simulink model "Aenea_model"  (R2020b)
settings: Solver=FixedStepDiscrete  StartTime=0.0  StopTime=10.0  FixedStep=0.02  RelTol=1e-3
values from neighbouring files (symbols this model uses):
  attuatore_Amax = deg2rad(27)    [AVVIO_AENEA_DATA.m]
  attuatore_Amin = deg2rad(-23)    [AVVIO_AENEA_DATA.m]
  attuatore_Emax = deg2rad(18)    [AVVIO_AENEA_DATA.m]
  attuatore_Emin = deg2rad(-32)    [AVVIO_AENEA_DATA.m]
  attuatore_Rmax = deg2rad(30)    [AVVIO_AENEA_DATA.m]
  attuatore_Rmin = deg2rad(-30)    [AVVIO_AENEA_DATA.m]
  attuatore_Tmax = 1    [AVVIO_AENEA_DATA.m]
  attuatore_Tmin = 0    [AVVIO_AENEA_DATA.m]
  interventoA_05 = 25    [AVVIO_AENEA_DATA.m]
  interventoA_1 = 20    [AVVIO_AENEA_DATA.m]
  interventoE_05 = 20    [AVVIO_AENEA_DATA.m]
  interventoE_1 = 15    [AVVIO_AENEA_DATA.m]
  interventoT = 0.1    [AVVIO_AENEA_DATA.m]
  inv_A = -1    [AVVIO_AENEA_DATA.m]
  inv_comp_h = -1    [AVVIO_AENEA_DATA.m]
  inv_E = 1    [AVVIO_AENEA_DATA.m]
  inv_R = 1    [AVVIO_AENEA_DATA.m]
  inv_T = 1    [AVVIO_AENEA_DATA.m]
  K_AW_B_AP_quota = 1000    [AVVIO_AENEA_DATA.m]
  K_AW_B_becc = -250    [AVVIO_AENEA_DATA.m]
  K_AW_B_imb = 0    [AVVIO_AENEA_DATA.m]
  K_AW_B_roll = 500    [AVVIO_AENEA_DATA.m]
  K_imb_inv = -1    [AVVIO_AENEA_DATA.m]
  Kd_h_app = 0.085    [AVVIO_AENEA_DATA.m]
  Kd_h_flare = 0.01    [AVVIO_AENEA_DATA.m]
  Ki_AP_quota_select = 0.014    [AVVIO_AENEA_DATA.m]
  Ki_AP_rotta = 0.03    [AVVIO_AENEA_DATA.m]
  Ki_AP_vel = 0.001*8    (= 0.008)    [AVVIO_AENEA_DATA.m]
  Ki_becch = -0.064065*10    (= -0.64065)    [AVVIO_AENEA_DATA.m]
  Ki_h_app = 0.055    [AVVIO_AENEA_DATA.m]
  Ki_h_cruise = 0.008    [AVVIO_AENEA_DATA.m]
  Ki_h_flare = 0.07    [AVVIO_AENEA_DATA.m]
  Ki_roll = 0.025*10    (= 0.25)    [AVVIO_AENEA_DATA.m]
  Kp_AP_quota_hold_h = 0.15    [AVVIO_AENEA_DATA.m]
  Kp_AP_quota_hold_l = 1    [AVVIO_AENEA_DATA.m]
  Kp_AP_quota_select = 0.014    [AVVIO_AENEA_DATA.m]
  Kp_AP_rotta = 0.7    [AVVIO_AENEA_DATA.m]
  Kp_AP_vel = 0.2692/8    (= 0.03365)    [AVVIO_AENEA_DATA.m]
  Kp_becch = -0.1918*10    (= -1.918)    [AVVIO_AENEA_DATA.m]
  Kp_comp_h = 0.035*15    (= 0.525)    [AVVIO_AENEA_DATA.m]
  Kp_h_app_max = 0.086    [AVVIO_AENEA_DATA.m]
  Kp_h_app_min = 0.01    [AVVIO_AENEA_DATA.m]
  Kp_h_cruise = 0.04    [AVVIO_AENEA_DATA.m]
  Kp_h_flare = 0.1    [AVVIO_AENEA_DATA.m]
  Kp_imb = -0.04*10    (= -0.4)    [AVVIO_AENEA_DATA.m]
  Kp_p = 0.025*5    (= 0.125)    [AVVIO_AENEA_DATA.m]
  Kp_q = -0.025*5    (= -0.125)    [AVVIO_AENEA_DATA.m]
  Kp_roll = 0.11*10    (= 1.1)    [AVVIO_AENEA_DATA.m]
  Kp_Rotta_ATO = 4    [AVVIO_AENEA_DATA.m]
  phi_max = deg2rad(30)    [AVVIO_AENEA_DATA.m]
  phi_min = deg2rad(-30)    [AVVIO_AENEA_DATA.m]
  pwm_aileron_max = 1940    [AVVIO_AENEA_DATA.m]
  pwm_aileron_min = 1099    [AVVIO_AENEA_DATA.m]
  pwm_elevator_max = 1939    [AVVIO_AENEA_DATA.m]
  pwm_elevator_min = 1099    [AVVIO_AENEA_DATA.m]
  pwm_rudder_max = 1971    [AVVIO_AENEA_DATA.m]
  pwm_rudder_min = 1130    [AVVIO_AENEA_DATA.m]
  pwm_throttle_max = 1940    [AVVIO_AENEA_DATA.m]
  pwm_throttle_min = 1160    [AVVIO_AENEA_DATA.m]
  safe_phi = 55    [AVVIO_AENEA_DATA.m]
  safe_V = 40    [AVVIO_AENEA_DATA.m]
  t_AP = 0.02    [AVVIO_AENEA_DATA.m]
  theta_max = deg2rad(15)    [AVVIO_AENEA_DATA.m]
  theta_min = deg2rad(-15)    [AVVIO_AENEA_DATA.m]
  time_alarm_SAFE = 1    [AVVIO_AENEA_DATA.m]
  V_max = 30    [AVVIO_AENEA_DATA.m]
  V_stall = 11    [AVVIO_AENEA_DATA.m]
  vel_wp1_al = 25    [AVVIO_AENEA_DATA.m]
  vel_wp2_al = 20    [AVVIO_AENEA_DATA.m]
undefined symbols (not defined in the file or in its folder): bias, DiscIntNeverNeededParam, Newton, Q1B, R1B, Raphson, Sensor_Offsets, tsamp, UP, vd_ini
libraries: simulink_extras x41, slpidlib x8, simulink x6, dspsigops x4, arduinolib x3, svdutilitieslib x3, aerolibtransform2sys x2, aerolibtransform2 x2, aerosimlib x2, cstblocks x1
(part 2 of 8)

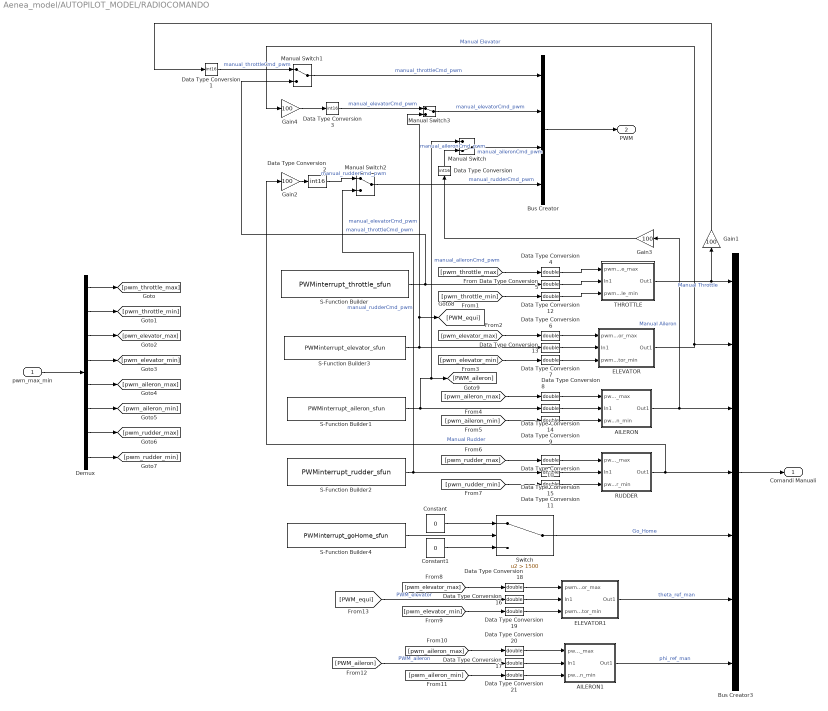
== system Aenea_model/AUTOPILOT_MODEL/RADIOCOMANDO ==
  pwm_max_min : Inport
  AILERON : Subsystem
  AILERON1 : Subsystem
  Bus Creator : BusCreator  Inputs=4
  Bus Creator3 : BusCreator  Inputs=7
  Constant : Constant  Value=0
  Constant1 : Constant  Value=0
  Data Type Conversion{,1..3} (4 alike) : DataTypeConversion  OutDataTypeStr=int16
  Data Type Conversion{4..21} (18 alike) : DataTypeConversion  OutDataTypeStr=double
  Demux : Demux  Outputs=8
  ELEVATOR : Subsystem
  ELEVATOR1 : Subsystem
  Gain{1..4} (4 alike) : Gain  Gain=100
  Manual Switch : ManualSwitch  CurrentSetting=0
  Manual Switch1 : ManualSwitch
  Manual Switch2 : ManualSwitch
  Manual Switch3 : ManualSwitch
  RUDDER : Subsystem
  S-Function Builder : S-Function  FunctionName=PWMinterrupt_throttle_sfun  SFunctionModules=PWMinterrupt_throttle_sfun_wrapper  SFunctionDeploymentMode=off  EnableBusSupport=off  mask(S-Function Builder){}
      mask help: Simulink:masks:SFunctionBuilder_MD
      mask init: same as Aenea_model/LOG_DATA_MODEL/S-Function Builder
      settings: CopyFcn=set_param(gcbh,'LinkStatus','none')  OpenFcn=sfunctionwizard(gcbh)
      mask Display: plot(val(:,1),val(:,2)),disp(sys),port_label('output',1,'out')
  S-Function Builder1 : S-Function  FunctionName=PWMinterrupt_aileron_sfun  SFunctionModules=PWMinterrupt_aileron_sfun_wrapper  SFunctionDeploymentMode=off  EnableBusSupport=off  mask(S-Function Builder){}
      mask help: Simulink:masks:SFunctionBuilder_MD
      mask init: same as Aenea_model/LOG_DATA_MODEL/S-Function Builder
      settings: CopyFcn=set_param(gcbh,'LinkStatus','none')  OpenFcn=sfunctionwizard(gcbh)
      mask Display: plot(val(:,1),val(:,2)),disp(sys),port_label('output',1,'out')
  S-Function Builder2 : S-Function  FunctionName=PWMinterrupt_rudder_sfun  SFunctionModules=PWMinterrupt_rudder_sfun_wrapper  SFunctionDeploymentMode=off  EnableBusSupport=off  mask(S-Function Builder){}
      mask help: Simulink:masks:SFunctionBuilder_MD
      mask init: same as Aenea_model/LOG_DATA_MODEL/S-Function Builder
      settings: CopyFcn=set_param(gcbh,'LinkStatus','none')  OpenFcn=sfunctionwizard(gcbh)
      mask Display: plot(val(:,1),val(:,2)),disp(sys),port_label('output',1,'out')
  S-Function Builder3 : S-Function  FunctionName=PWMinterrupt_elevator_sfun  SFunctionModules=PWMinterrupt_elevator_sfun_wrapper  SFunctionDeploymentMode=off  EnableBusSupport=off  mask(S-Function Builder){}
      mask help: Simulink:masks:SFunctionBuilder_MD
      mask init: same as Aenea_model/LOG_DATA_MODEL/S-Function Builder
      settings: CopyFcn=set_param(gcbh,'LinkStatus','none')  OpenFcn=sfunctionwizard(gcbh)
      mask Display: plot(val(:,1),val(:,2)),disp(sys),port_label('output',1,'out')
  S-Function Builder4 : S-Function  FunctionName=PWMinterrupt_goHome_sfun  SFunctionModules=PWMinterrupt_goHome_sfun_wrapper  SFunctionDeploymentMode=off  EnableBusSupport=off  mask(S-Function Builder){}
      mask help: Simulink:masks:SFunctionBuilder_MD
      mask init: same as Aenea_model/LOG_DATA_MODEL/S-Function Builder
      settings: CopyFcn=set_param(gcbh,'LinkStatus','none')  OpenFcn=sfunctionwizard(gcbh)
      mask Display: plot(val(:,1),val(:,2)),disp(sys),port_label('output',1,'out')
  Switch : Switch  Criteria=u2 > Threshold  Threshold=1500
  THROTTLE : Subsystem
  Comandi Manuali : Outport  VectorParamsAs1DForOutWhenUnconnected=off
  PWM : Outport  Port=2  VectorParamsAs1DForOutWhenUnconnected=off
  wires:
  Bus Creator3/1 -> Comandi Manuali/1
  S-Function Builder4/1 -> Switch/2
  Constant/1 -> Switch/1
  Constant1/1 -> Switch/3
  Switch/1 -> Bus Creator3/5  "Go_Home"
  S-Function Builder2/1 -> Manual Switch2/2, Data Type Conversion15/1  "manual_rudderCmd_pwm"
  S-Function Builder3/1 -> Manual Switch3/2, [PWM_equi], Data Type Conversion13/1  "manual_elevatorCmd_pwm"
  S-Function Builder1/1 -> Data Type Conversion14/1, Manual Switch/1, [PWM_aileron]  "manual_aileronCmd_pwm"
  S-Function Builder/1 -> Manual Switch1/2, Data Type Conversion5/1  "manual_throttleCmd_pwm"
  THROTTLE/1(Out1) -> Gain1/1, Bus Creator3/1  "Manual Throttle"
  ELEVATOR/1(Out1) -> Bus Creator3/2, Gain4/1  "Manual Elevator"
  AILERON/1(Out1) -> Gain3/1, Bus Creator3/3  "Manual Aileron"
  RUDDER/1(Out1) -> Bus Creator3/4, Gain2/1  "Manual Rudder"
  Bus Creator/1 -> PWM/1
  pwm_max_min/1 -> Demux/1
  Demux/1 -> [pwm_throttle_max]
  Demux/2 -> [pwm_throttle_min]
  Demux/3 -> [pwm_elevator_max]
  Demux/4 -> [pwm_elevator_min]
  Demux/5 -> [pwm_aileron_max]
  Demux/6 -> [pwm_aileron_min]
  Demux/8 -> [pwm_rudder_min]
  Demux/7 -> [pwm_rudder_max]
  [pwm_elevator_min] -> Data Type Conversion7/1
  [pwm_elevator_max] -> Data Type Conversion6/1
  [pwm_aileron_min] -> Data Type Conversion9/1
  [pwm_aileron_max] -> Data Type Conversion8/1
  [pwm_rudder_max] -> Data Type Conversion10/1
  [pwm_rudder_min] -> Data Type Conversion11/1
  [pwm_throttle_max] -> Data Type Conversion4/1
  [pwm_throttle_min] -> Data Type Conversion12/1
  Data Type Conversion6/1 -> ELEVATOR/1(pwm_elevator_max)
  Data Type Conversion7/1 -> ELEVATOR/3(pwm_elevator_min)
  Data Type Conversion8/1 -> AILERON/1(pwm_aileron_max)
  Data Type Conversion9/1 -> AILERON/3(pwm_aileron_min)
  Data Type Conversion10/1 -> RUDDER/1(pwm_rudder_max)
  Data Type Conversion11/1 -> RUDDER/3(pwm_rudder_min)
  Data Type Conversion4/1 -> THROTTLE/1(pwm_throttle_max)
  Data Type Conversion5/1 -> THROTTLE/2(In1)
  Data Type Conversion12/1 -> THROTTLE/3(pwm_throttle_min)
  Data Type Conversion13/1 -> ELEVATOR/2(In1)
  Data Type Conversion14/1 -> AILERON/2(In1)
  Data Type Conversion15/1 -> RUDDER/2(In1)
  [pwm_aileron_max] -> Data Type Conversion20/1
  AILERON1/1(Out1) -> Bus Creator3/7  "phi_ref_man"
  [PWM_equi] -> Data Type Conversion16/1  "PWM_elevator"
  ELEVATOR1/1(Out1) -> Bus Creator3/6  "theta_ref_man"
  [pwm_elevator_min] -> Data Type Conversion19/1
  Data Type Conversion17/1 -> AILERON1/2(In1)
  [pwm_aileron_min] -> Data Type Conversion21/1
  Data Type Conversion21/1 -> AILERON1/3(pwm_aileron_min)
  Data Type Conversion18/1 -> ELEVATOR1/1(pwm_elevator_max)
  Data Type Conversion16/1 -> ELEVATOR1/2(In1)
  Data Type Conversion20/1 -> AILERON1/1(pwm_aileron_max)
  Data Type Conversion19/1 -> ELEVATOR1/3(pwm_elevator_min)
  [pwm_elevator_max] -> Data Type Conversion18/1
  [PWM_aileron] -> Data Type Conversion17/1  "PWM_aileron"
  Gain3/1 -> Data Type Conversion/1
  Data Type Conversion/1 -> Manual Switch/2  "manual_aileronCmd_pwm"
  Gain4/1 -> Data Type Conversion3/1
  Data Type Conversion3/1 -> Manual Switch3/1  "manual_elevatorCmd_pwm"
  Data Type Conversion1/1 -> Manual Switch1/1  "manual_throttleCmd_pwm"
  Gain1/1 -> Data Type Conversion1/1
  Gain2/1 -> Data Type Conversion2/1
  Data Type Conversion2/1 -> Manual Switch2/1  "manual_rudderCmd_pwm"
  Manual Switch/1 -> Bus Creator/3  "manual_aileronCmd_pwm"
  Manual Switch1/1 -> Bus Creator/1  "manual_throttleCmd_pwm"
  Manual Switch2/1 -> Bus Creator/4  "manual_rudderCmd_pwm"
  Manual Switch3/1 -> Bus Creator/2  "manual_elevatorCmd_pwm"

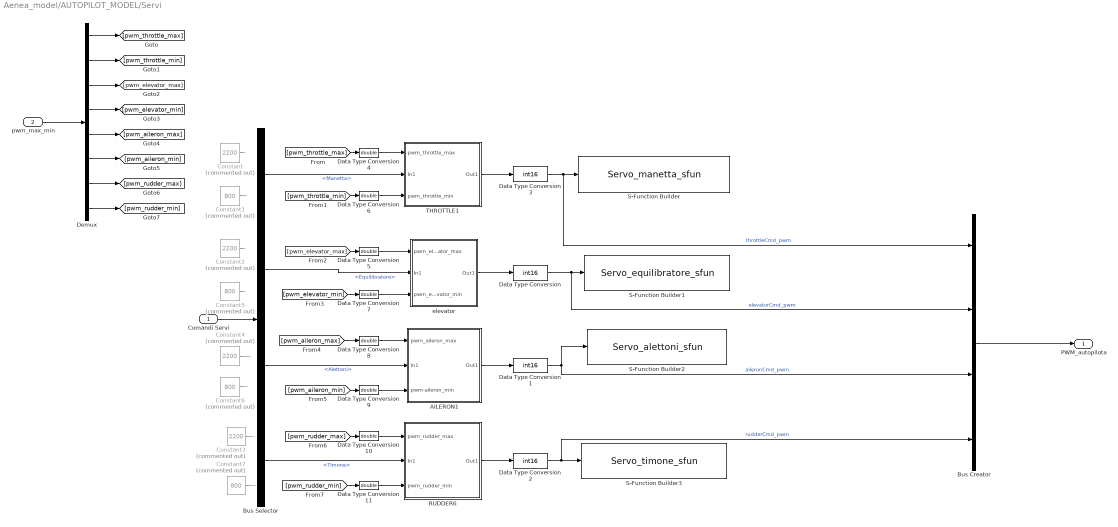
== system Aenea_model/AUTOPILOT_MODEL/Servi ==
  Comandi Servi : Inport
  pwm_max_min : Inport  Port=2
  AILERON1 : Subsystem
  Bus Creator : BusCreator  Inputs=4
  Bus Selector : BusSelector  OutputSignals=Manetta,Equilibratore,Alettoni,Timone
  Constant{,2..4} (4 alike) : Constant  Commented=on  Value=2200
  Constant{1,5..7} (4 alike) : Constant  Commented=on  Value=800
  Data Type Conversion{,1..3} (4 alike) : DataTypeConversion  OutDataTypeStr=int16
  Data Type Conversion{4..11} (8 alike) : DataTypeConversion  OutDataTypeStr=double
  Demux : Demux  Outputs=8
  RUDDER6 : Subsystem
  S-Function Builder : S-Function  FunctionName=Servo_manetta_sfun  SFunctionModules=Servo_manetta_sfun_wrapper  SFunctionDeploymentMode=off  EnableBusSupport=off  mask(S-Function Builder){}
      mask help: Simulink:masks:SFunctionBuilder_MD
      mask init: same as Aenea_model/LOG_DATA_MODEL/S-Function Builder
      settings: CopyFcn=set_param(gcbh,'LinkStatus','none')  OpenFcn=sfunctionwizard(gcbh)
      mask Display:
      | plot(val(:,1),val(:,2))
      | disp(sys)
      | port_label('input',1,'tau')
  S-Function Builder1 : S-Function  FunctionName=Servo_equilibratore_sfun  SFunctionModules=Servo_equilibratore_sfun_wrapper  SFunctionDeploymentMode=off  EnableBusSupport=off  mask(S-Function Builder){}
      mask help: Simulink:masks:SFunctionBuilder_MD
      mask init: same as Aenea_model/LOG_DATA_MODEL/S-Function Builder
      settings: CopyFcn=set_param(gcbh,'LinkStatus','none')  OpenFcn=sfunctionwizard(gcbh)
      mask Display:
      | plot(val(:,1),val(:,2))
      | disp(sys)
      | port_label('input',1,'tau')
  S-Function Builder2 : S-Function  FunctionName=Servo_alettoni_sfun  SFunctionModules=Servo_alettoni_sfun_wrapper  SFunctionDeploymentMode=off  EnableBusSupport=off  mask(S-Function Builder){}
      mask help: Simulink:masks:SFunctionBuilder_MD
      mask init: same as Aenea_model/LOG_DATA_MODEL/S-Function Builder
      settings: CopyFcn=set_param(gcbh,'LinkStatus','none')  OpenFcn=sfunctionwizard(gcbh)
      mask Display:
      | plot(val(:,1),val(:,2))
      | disp(sys)
      | port_label('input',1,'tau')
  S-Function Builder3 : S-Function  FunctionName=Servo_timone_sfun  SFunctionModules=Servo_timone_sfun_wrapper  SFunctionDeploymentMode=off  EnableBusSupport=off  mask(S-Function Builder){}
      mask help: Simulink:masks:SFunctionBuilder_MD
      mask init: same as Aenea_model/LOG_DATA_MODEL/S-Function Builder
      settings: CopyFcn=set_param(gcbh,'LinkStatus','none')  OpenFcn=sfunctionwizard(gcbh)
      mask Display:
      | plot(val(:,1),val(:,2))
      | disp(sys)
      | port_label('input',1,'tau')
  THROTTLE1 : Subsystem
  elevator : Subsystem
  PWM_autopilota : Outport  VectorParamsAs1DForOutWhenUnconnected=off
  wires:
  AILERON1/1(Out1) -> Data Type Conversion1/1
  THROTTLE1/1(Out1) -> Data Type Conversion3/1
  RUDDER6/1(Out1) -> Data Type Conversion2/1
  elevator/1(Out1) -> Data Type Conversion/1
  Bus Selector/1 -> THROTTLE1/2(In1)  "<Manetta>"
  Bus Selector/4 -> RUDDER6/2(In1)  "<Timone>"
  Bus Selector/3 -> AILERON1/2(In1)  "<Alettoni>"
  Bus Selector/2 -> elevator/2(In1)  "<Equilibratore>"
  Comandi Servi/1 -> Bus Selector/1
  Demux/3 -> [pwm_elevator_max]
  Demux/2 -> [pwm_throttle_min]
  Demux/6 -> [pwm_aileron_min]
  Demux/1 -> [pwm_throttle_max]
  Demux/8 -> [pwm_rudder_min]
  Demux/7 -> [pwm_rudder_max]
  Demux/5 -> [pwm_aileron_max]
  Demux/4 -> [pwm_elevator_min]
  [pwm_throttle_max] -> Data Type Conversion4/1
  [pwm_throttle_min] -> Data Type Conversion6/1
  [pwm_elevator_max] -> Data Type Conversion5/1
  [pwm_elevator_min] -> Data Type Conversion7/1
  [pwm_aileron_max] -> Data Type Conversion8/1
  [pwm_aileron_min] -> Data Type Conversion9/1
  [pwm_rudder_max] -> Data Type Conversion10/1
  Data Type Conversion/1 -> S-Function Builder1/1, Bus Creator/2  "elevatorCmd_pwm"
  Data Type Conversion1/1 -> S-Function Builder2/1, Bus Creator/3  "aileronCmd_pwm"
  Data Type Conversion3/1 -> S-Function Builder/1, Bus Creator/1  "throttleCmd_pwm"
  Data Type Conversion2/1 -> S-Function Builder3/1, Bus Creator/4  "rudderCmd_pwm"
  Data Type Conversion4/1 -> THROTTLE1/1(pwm_throttle_max)
  Data Type Conversion6/1 -> THROTTLE1/3(pwm_throttle_min)
  Data Type Conversion5/1 -> elevator/1(pwm_elevator_max)
  Data Type Conversion7/1 -> elevator/3(pwm_elevator_min)
  Data Type Conversion8/1 -> AILERON1/1(pwm_aileron_max)
  Data Type Conversion9/1 -> AILERON1/3(pwm-aileron_min)
  Data Type Conversion10/1 -> RUDDER6/1(pwm_rudder_max)
  Data Type Conversion11/1 -> RUDDER6/3("pwm_rudder_min ")
  Bus Creator/1 -> PWM_autopilota/1
  Constant1/1 -> ?
  Constant/1 -> ?
  Constant2/1 -> ?
  Constant3/1 -> ?
  Constant4/1 -> ?
  Constant5/1 -> ?
  Constant6/1 -> ?
  Constant7/1 -> ?
  pwm_max_min/1 -> Demux/1
  [pwm_rudder_min] -> Data Type Conversion11/1

== system Aenea_model/LOG_DATA_MODEL/LOG_BOOL_SIGNALS ==
  dummy16 : Inport
  Bus Creator11 : BusCreator  Inputs=2  OutDataTypeStr=Bus: BUS_bool_log_t  NonVirtualBus=on
      settings: InheritFromInputs=off
  Constant24 : Constant  Value=true  OutDataTypeStr=boolean
  bool_data : Outport
  wires:
  Constant24/1 -> Bus Creator11/1  "dummy12"
  Bus Creator11/1 -> bool_data/1  "bool_data"
  dummy16/1 -> Bus Creator11/2

== system Aenea_model/LOG_DATA_MODEL/LOG_DOUBLE_SIGNALS ==
  double_in : Inport
  Bus Creator : BusCreator  Inputs=8
  Bus Selector : BusSelector  OutputSignals=sensor_data_raw.Lat,sensor_data_raw.Long,sensor_data_filtered.Lat,sensor_data_filtered.Long,absDelta.absE,absDelta.absA,absDelta.absT
  Mux : Mux  Inputs=1
  Mux1 : Mux  Inputs=1
  Radians to Degrees : simulink_extras/Transformations/Radians to Degrees
  Radians to Degrees1 : simulink_extras/Transformations/Radians to Degrees
  Subsystem : Subsystem
  double_data : Outport
  wires:
  Bus Creator/1 -> double_data/1  "double_data"
  Subsystem/1(frame_count) -> Bus Creator/1  "time_frame"
  double_in/1 -> Bus Selector/1
  Bus Selector/1 -> Mux/1  "<Lat>"
  Bus Selector/2 -> Mux1/1  "<Long>"
  Bus Selector/3 -> Radians to Degrees/1  "<Lat>"
  Bus Selector/4 -> Radians to Degrees1/1  "<Long>"
  Mux/1 -> Bus Creator/2  "Lat_raw"
  Mux1/1 -> Bus Creator/3  "Long_raw"
  Radians to Degrees/1 -> Bus Creator/4  "Lat"
  Radians to Degrees1/1 -> Bus Creator/5  "Long"
  Bus Selector/5 -> Bus Creator/6  "<absE>"
  Bus Selector/6 -> Bus Creator/7  "<absA>"
  Bus Selector/7 -> Bus Creator/8  "<absT>"

== system Aenea_model/LOG_DATA_MODEL/LOG_INT16_SIGNALS ==
  int16_in : Inport
  Bus Creator7 : BusCreator  Inputs=8  OutDataTypeStr=Bus: BUS_int16_log_t  NonVirtualBus=on
      settings: InheritFromInputs=off
  Bus Selector : BusSelector  OutputSignals=sensor_data_raw.Comandi.manual_throttleCmd_pwm,sensor_data_raw.Comandi.manual_elevatorCmd_pwm,sensor_data_raw.Comandi.manual_aileronCmd_pwm,sensor_data_raw.Comandi.manual_rudderCmd_pwm,sensor_data_raw.PWM_autopilota.throttleCmd_pwm,sensor_data_raw.PWM_autopilota.elevatorCmd_pwm,sensor_data_raw.PWM_autopilota.aileronCmd_pwm,sensor_data_raw.PWM_autopilota.rudderCmd_pwm
  int16_data : Outport
  wires:
  Bus Creator7/1 -> int16_data/1  "int16_data"
  int16_in/1 -> Bus Selector/1
  Bus Selector/1 -> Bus Creator7/1  "<manual_throttleCmd_pwm>"
  Bus Selector/2 -> Bus Creator7/2  "<manual_elevatorCmd_pwm>"
  Bus Selector/3 -> Bus Creator7/3  "<manual_aileronCmd_pwm>"
  Bus Selector/4 -> Bus Creator7/4  "<manual_rudderCmd_pwm>"
  Bus Selector/5 -> Bus Creator7/5  "<throttleCmd_pwm>"
  Bus Selector/6 -> Bus Creator7/6  "<elevatorCmd_pwm>"
  Bus Selector/7 -> Bus Creator7/7  "<aileronCmd_pwm>"
  Bus Selector/8 -> Bus Creator7/8  "<rudderCmd_pwm>"

== system Aenea_model/LOG_DATA_MODEL/LOG_INT32_SIGNALS ==
  Bus Creator5 : BusCreator  Inputs=2  OutDataTypeStr=Bus: BUS_int32_log_t  NonVirtualBus=on
      settings: InheritFromInputs=off
  Constant18 : Constant  Value=-15  OutDataTypeStr=int32
  Constant9 : Constant  Value=528  OutDataTypeStr=int32
  int32_data : Outport
  wires:
  Constant18/1 -> Bus Creator5/2  "dummy4"
  Bus Creator5/1 -> int32_data/1  "int32_data"
  Constant9/1 -> Bus Creator5/1  "dummy3"

== system Aenea_model/LOG_DATA_MODEL/LOG_INT8_SIGNALS ==
  IN_LOG : Inport
  Bus Creator9 : BusCreator  Inputs=2  OutDataTypeStr=Bus: BUS_int8_log_t  NonVirtualBus=on
      settings: InheritFromInputs=off
  Bus Selector : BusSelector  OutputSignals=modo.modo,go_home
  Data Type Conversion : DataTypeConversion  OutDataTypeStr=int8
  Data Type Conversion1 : DataTypeConversion  OutDataTypeStr=int8
  int8_data : Outport
  wires:
  IN_LOG/1 -> Bus Selector/1
  Bus Creator9/1 -> int8_data/1  "int8_data"
  Bus Selector/1 -> Data Type Conversion/1  "<modo>"
  Data Type Conversion/1 -> Bus Creator9/1
  Bus Selector/2 -> Data Type Conversion1/1  "<go_home>"
  Data Type Conversion1/1 -> Bus Creator9/2

== system Aenea_model/LOG_DATA_MODEL/LOG_SINGLE_SIGNALS ==
  single_in : Inport
  Bus Creator4 : BusCreator  Inputs=24  OutDataTypeStr=Bus: BUS_single_log_t  NonVirtualBus=on
      settings: InheritFromInputs=off
  Bus Selector : BusSelector  OutputSignals=sensor_data_raw.V_GPS,sensor_data_raw.quota_GPS,sensor_data_raw.heading,sensor_data_raw.acc x,sensor_data_raw.acc y,sensor_data_raw.acc z,sensor_data_raw.p,sensor_data_raw.q,sensor_data_raw.r,sensor_data_raw.phi,sensor_data_raw.theta,sensor_data_raw.psi,sensor_data_raw.V_pitot,sensor_data_raw.dist_lidar,sensor_data_raw.quota_baro,sensor_data_raw.pressione,sensor_data_raw.temperatura,sensor_data_filtered.Alt,sensor_data_filtered.ias,sensor_data_filtered.RC,sensor_data_filtered.horiz_speed,sensor_data_filtered.heading,sensor_data_filtered.quota_lidar,dp
  Data Type Conversion{,1..23} (24 alike) : DataTypeConversion  OutDataTypeStr=single
  single_data : Outport
  wires:
  Bus Creator4/1 -> single_data/1  "single_data"
  single_in/1 -> Bus Selector/1
  Bus Selector/2 -> Data Type Conversion1/1  "<quota_GPS>"
  Bus Selector/1 -> Data Type Conversion/1  "<V_GPS>"
  Bus Selector/3 -> Data Type Conversion2/1  "<heading>"
  Bus Selector/4 -> Data Type Conversion3/1  "<acc x>"
  Bus Selector/5 -> Data Type Conversion4/1  "<acc y>"
  Bus Selector/6 -> Data Type Conversion5/1  "<acc z>"
  Bus Selector/7 -> Data Type Conversion6/1  "<p>"
  Bus Selector/8 -> Data Type Conversion7/1  "<q>"
  Bus Selector/9 -> Data Type Conversion8/1  "<r>"
  Bus Selector/11 -> Data Type Conversion9/1  "<theta>"
  Bus Selector/12 -> Data Type Conversion10/1  "<psi>"
  Bus Selector/13 -> Data Type Conversion11/1  "<V_pitot>"
  Bus Selector/14 -> Data Type Conversion12/1  "<dist_lidar>"
  Data Type Conversion/1 -> Bus Creator4/1  "v_gps_raw"
  Data Type Conversion1/1 -> Bus Creator4/2  "h_gps_raw"
  Data Type Conversion2/1 -> Bus Creator4/3  "heading_raw"
  Data Type Conversion3/1 -> Bus Creator4/4  "acc_x_raw"
  Data Type Conversion5/1 -> Bus Creator4/6  "acc_z_raw"
  Data Type Conversion6/1 -> Bus Creator4/7  "p_raw"
  Data Type Conversion7/1 -> Bus Creator4/8  "q_raw"
  Data Type Conversion4/1 -> Bus Creator4/5  "acc_y_raw"
  Data Type Conversion8/1 -> Bus Creator4/9  "r_raw"
  Data Type Conversion10/1 -> Bus Creator4/12  "psi_raw"
  Data Type Conversion9/1 -> Bus Creator4/11  "theta_raw"
  Data Type Conversion11/1 -> Bus Creator4/13  "v_pitot_raw"
  Data Type Conversion12/1 -> Bus Creator4/14  "dist_lidar_raw"
  Bus Selector/10 -> Data Type Conversion13/1  "<phi>"
  Data Type Conversion13/1 -> Bus Creator4/10  "phi_raw"
  Bus Selector/18 -> Data Type Conversion18/1  "<Alt>"
  Bus Selector/19 -> Data Type Conversion17/1  "<ias>"
  Bus Selector/20 -> Data Type Conversion19/1  "<RC>"
  Bus Selector/21 -> Data Type Conversion14/1  "<horiz_speed>"
  Bus Selector/22 -> Data Type Conversion15/1  "<heading>"
  Bus Selector/23 -> Data Type Conversion16/1  "<quota_lidar>"
  Data Type Conversion18/1 -> Bus Creator4/18  "h_baro_filt"
  Data Type Conversion17/1 -> Bus Creator4/19  "ias_filt"
  Data Type Conversion19/1 -> Bus Creator4/20  "RC_filt"
  Data Type Conversion14/1 -> Bus Creator4/21  "groundspeed_filt"
  Data Type Conversion15/1 -> Bus Creator4/22  "heading_filt"
  Data Type Conversion16/1 -> Bus Creator4/23  "dist_lidar_filt"
  Bus Selector/15 -> Data Type Conversion20/1  "<quota_baro>"
  Bus Selector/16 -> Data Type Conversion21/1  "<pressione>"
  Bus Selector/17 -> Data Type Conversion22/1  "<temperatura>"
  Data Type Conversion20/1 -> Bus Creator4/15  "h_baro_raw"
  Data Type Conversion21/1 -> Bus Creator4/16  "press_raw"
  Data Type Conversion22/1 -> Bus Creator4/17  "temp_raw"
  Bus Selector/24 -> Data Type Conversion23/1  "<dp>"
  Data Type Conversion23/1 -> Bus Creator4/24  "dp_raw"

== system Aenea_model/LOG_DATA_MODEL/LOG_UINT16_SIGNALS ==
  Bus Creator8 : BusCreator  Inputs=2  OutDataTypeStr=Bus: BUS_uint16_log_t  NonVirtualBus=on
      settings: InheritFromInputs=off
  Constant11 : Constant  Value=20  OutDataTypeStr=uint16
  Constant22 : Constant  Value=20  OutDataTypeStr=uint16
  uint16_data : Outport
  wires:
  Bus Creator8/1 -> uint16_data/1  "uint16_data"
  Constant22/1 -> Bus Creator8/2  "dummy10"
  Constant11/1 -> Bus Creator8/1  "dummy9"

== system Aenea_model/LOG_DATA_MODEL/LOG_UINT32_SIGNALS ==
  Bus Creator6 : BusCreator  Inputs=2  OutDataTypeStr=Bus: BUS_uint32_log_t  NonVirtualBus=on
      settings: InheritFromInputs=off
  Constant19 : Constant  Value=15  OutDataTypeStr=uint32
  Constant20 : Constant  Value=1078  OutDataTypeStr=uint32
  uint32_data : Outport
  wires:
  Constant20/1 -> Bus Creator6/2  "dummy6"
  Constant19/1 -> Bus Creator6/1  "dummy5"
  Bus Creator6/1 -> uint32_data/1  "uint32_data"

== system Aenea_model/LOG_DATA_MODEL/LOG_UINT8_SIGNALS ==
  uint8_in : Inport
  Bus Creator : BusCreator  Inputs=2
  Bus Selector : BusSelector  OutputSignals=sensor_data_raw.fix,Base_mode
  Data Type Conversion : DataTypeConversion  OutDataTypeStr=uint8
  Data Type Conversion1 : DataTypeConversion  OutDataTypeStr=uint8
  uint8_data : Outport
  wires:
  Data Type Conversion/1 -> Bus Creator/1  "gps_fix"
  uint8_in/1 -> Bus Selector/1
  Bus Creator/1 -> uint8_data/1  "uint8_data"
  Bus Selector/1 -> Data Type Conversion/1  "<fix>"
  Bus Selector/2 -> Data Type Conversion1/1  "<Base_mode>"
  Data Type Conversion1/1 -> Bus Creator/2  "Base_mode"

== system Aenea_model/AUTOPILOT_MODEL/AIR TX/Enable  ==
  In1 : Inport
  In2 : Inport  Port=2
  Enable : EnablePort
  Chart : Stateflow chart  TreatAsAtomicUnit=on
  wires:
  In2/1 -> Chart/2(Len)
  In1/1 -> Chart/1(datain)

== system Aenea_model/AUTOPILOT_MODEL/AIR TX/GPS ==
  note: NB.: se non si posside un dato inserire una costante con valore 0. I dati vanno messi tutti anche se zeri nell'ordine elencato
  note: Vanno inseriti i collegamenti con i dati provenienti dal sensore GPS
      | in uscita bisogna dare 3 segnali:
      |
      | -LLAA: latitudine, longitudine, altitudine, altitudine relativa
      | -VEL: velocità (x,y,z)
      | -HDG: heading
  GPS1 : Inport
  Bus Selector : BusSelector  OutputSignals=Lat,Long,Alt,horiz_speed,RC,heading
  Data Type Conversion : DataTypeConversion  OutDataTypeStr=int32  RndMeth=Simplest
  Data Type Conversion1 : DataTypeConversion  OutDataTypeStr=int16  RndMeth=Simplest
  Data Type Conversion2 : DataTypeConversion  OutDataTypeStr=uint16  RndMeth=Simplest
  Gain : Gain  Gain=[10^7;10^7;1000 ;1000]
  Gain1 : Gain  Gain=1000
  Gain2 : Gain  Gain=100
  Mux : Mux
  Mux1 : Mux  Inputs=3
  Radians to Degrees : simulink_extras/Transformations/Radians to Degrees
  Radians to Degrees2 : simulink_extras/Transformations/Radians to Degrees
  alt_r : Constant  Value=0
  vel y : Constant  Value=0  OutDataTypeStr=double
  LLAA : Outport  VectorParamsAs1DForOutWhenUnconnected=off
  vel : Outport  Port=2  VectorParamsAs1DForOutWhenUnconnected=off
  hdg1 : Outport  Port=3  VectorParamsAs1DForOutWhenUnconnected=off
  wires:
  Gain2/1 -> Data Type Conversion2/1
  Gain/1 -> Data Type Conversion/1
  Gain1/1 -> Data Type Conversion1/1
  Mux/1 -> Gain/1
  Bus Selector/6 -> Gain2/1  "<heading>"
  Bus Selector/5 -> Mux1/3  "<RC>"
  Mux1/1 -> Gain1/1  "VEL"
  alt_r/1 -> Mux/4
  GPS1/1 -> Bus Selector/1
  Bus Selector/1 -> Radians to Degrees/1  "<Lat>"
  Bus Selector/2 -> Radians to Degrees2/1  "<Long>"
  Bus Selector/4 -> Mux1/1  "<horiz_speed>"
  vel y/1 -> Mux1/2
  Data Type Conversion2/1 -> hdg1/1
  Data Type Conversion1/1 -> vel/1
  Data Type Conversion/1 -> LLAA/1
  Bus Selector/3 -> Mux/3  "<Alt>"
  Radians to Degrees/1 -> Mux/1  "Lat"
  Radians to Degrees2/1 -> Mux/2  "Long"

== system Aenea_model/AUTOPILOT_MODEL/AIR TX/Heartbeat ==
  note: Vanno inseriti i collegamenti con i dati provenienti dalla ricezione (stazione di terra) e gli allarmi
      | in uscita bisogna dare 2 vettori costituiti da:
      | -I:
      | -custom code (su può mettere ciò che si vuole)
      | -II:
      | -vettore di 2 componenti: tido di veivolo e tipo di autopilota
      | -vettore di due componenti che è creato tramite la matlabfuncition
  Alarm : Inport
  RX_mode : Inport  Port=2
  modo : Inport  Port=3
  Alarm set : MATLAB Function  TreatAsAtomicUnit=on
  Data Type Conversion : DataTypeConversion  OutDataTypeStr=uint32
  Data Type Conversion1 : DataTypeConversion  OutDataTypeStr=uint8
  Mux : Mux  Inputs=2
  Type fixed_wing Autopilot generic : Constant  Value=[1;0]  OutDataTypeStr=uint8
  custom : Outport  VectorParamsAs1DForOutWhenUnconnected=off
  H_data : Outport  Port=2  VectorParamsAs1DForOutWhenUnconnected=off
  wires:
  modo/1 -> Data Type Conversion/1
  Data Type Conversion1/1 -> H_data/1
  Data Type Conversion/1 -> custom/1
  RX_mode/1 -> Alarm set/2(Rx_mode)
  Alarm/1 -> Alarm set/1(Alarm)
  Type fixed_wing Autopilot generic/1 -> Mux/1
  Alarm set/1(H_mav) -> Mux/2
  Mux/1 -> Data Type Conversion1/1

== system Aenea_model/AUTOPILOT_MODEL/AIR TX/IMU & Attidude ==
  note: NB.: se non si posside un dato inserire una costante con valore 0. I dati vanno messi tutti anche se zeri nell'ordine elencato
  note: Vanno inseriti i collegamenti con i dati provenienti dal sensore inerziale (MTi)
      | in uscita bisogna dare un vettore di 12 componenti contente in ordine:
      | - 3 accelerazioni (x,y,z)
      | - 3 giroscopiche (p,q,r)
      | - 3 comp. campo magnetico
      | -3 angoli di eulero
  AHRS1 : Inport
  Bus Selector : BusSelector  OutputSignals=acc,p,q,r,phi,theta,psi
  Constant : Constant  Value=0  OutDataTypeStr=double  SampleTime=t_AP
  Constant1 : Constant  Value=0  OutDataTypeStr=double  SampleTime=t_AP
  Constant2 : Constant  Value=0  OutDataTypeStr=double  SampleTime=t_AP
  Data Type Conversion : DataTypeConversion  OutDataTypeStr=int16  RndMeth=Simplest
  Data Type Conversion1 : DataTypeConversion  OutDataTypeStr=single
  Gain : Gain  Gain=10^3
  Mux{1,3..5} (4 alike) : Mux  Inputs=3
  Mux2 : Mux  Inputs=2
  IMU : Outport  VectorParamsAs1DForOutWhenUnconnected=off
  ATT : Outport  Port=2  VectorParamsAs1DForOutWhenUnconnected=off
  wires:
  Constant/1 -> Mux5/1
  Mux4/1 -> Mux2/1
  Bus Selector/7 -> Mux4/3  "<psi>"
  Bus Selector/6 -> Mux4/2  "<theta>"
  Bus Selector/5 -> Mux4/1  "<phi>"
  Mux3/1 -> Mux2/2, Mux1/2
  Bus Selector/4 -> Mux3/3  "<r>"
  Bus Selector/3 -> Mux3/2  "<q>"
  Bus Selector/2 -> Mux3/1  "<p>"
  Bus Selector/1 -> Mux1/1  "<acc>"
  AHRS1/1 -> Bus Selector/1
  Mux2/1 -> Data Type Conversion1/1
  Gain/1 -> Data Type Conversion/1
  Data Type Conversion1/1 -> ATT/1
  Data Type Conversion/1 -> IMU/1
  Mux1/1 -> Gain/1
  Constant1/1 -> Mux5/2
  Mux5/1 -> Mux1/3
  Constant2/1 -> Mux5/3

== system Aenea_model/AUTOPILOT_MODEL/AIR TX/If_subsystem ==
  note: Blocco per la temporizzazione dell'invio dei messaggi
  Data Type Conversion3 : DataTypeConversion  OutDataTypeStr=uint32  RndMeth=Simplest
  Gain : Gain  Gain=100
  Subsystem : Subsystem
  iflogic_function : MATLAB Function  TreatAsAtomicUnit=on
  iflogic : Outport  VectorParamsAs1DForOutWhenUnconnected=off
  time : Outport  Port=2  VectorParamsAs1DForOutWhenUnconnected=off
  wires:
  Subsystem/3(time) -> Gain/1
  Subsystem/2(H_10) -> iflogic_function/2(H10)
  Subsystem/1(H_50) -> iflogic_function/1(H50)
  Gain/1 -> Data Type Conversion3/1
  Data Type Conversion3/1 -> time/1
  iflogic_function/1(iflogic) -> iflogic/1

== system Aenea_model/AUTOPILOT_MODEL/AIR TX/Servo ==
  note: NB.: se non si posside un dato inserire una costante con valore 0. I dati vanno messi tutti anche se zeri nell'ordine elencato
  note: Vanno inseriti i collegamenti con i dati provenienti dal sensore di velocità
      | in uscita bisogna dare 1 segnale composto da:
      |
      | -  PORT
      | -8 servo
  note: La quota lidar la invio come componente 8 dei servi
  Sensor : Inport
  Servo : Inport  Port=2
  Bus Selector : BusSelector  OutputSignals=Manetta,Equilibratore,Alettoni,Timone
  Bus Selector1 : BusSelector  OutputSignals=quota_lidar
  Constant : Constant  Value=4
  Constant1 : Constant  Value=zeros(3,1)
  Conversione : Subsystem
  Data Type Conversion1 : DataTypeConversion  OutDataTypeStr=uint16  RndMeth=Simplest
  Gain : Gain  Gain=100
  Mux : Mux  Inputs=7
  Saturation : Saturate  UpperLimit=4000  LowerLimit=0
  Servo_data : Outport  VectorParamsAs1DForOutWhenUnconnected=off
  wires:
  Conversione/4(Out4) -> Mux/5
  Conversione/3(Out3) -> Mux/4
  Conversione/2(Out2) -> Mux/3
  Conversione/1(Out1) -> Mux/2
  Bus Selector/1 -> Conversione/1(Manetta)  "<Manetta>"
  Bus Selector/4 -> Conversione/4(Timone)  "<Timone>"
  Bus Selector/3 -> Conversione/3(Alettoni)  "<Alettoni>"
  Bus Selector/2 -> Conversione/2(Equilibratore)  "<Equilibratore>"
  Constant1/1 -> Mux/6
  Constant/1 -> Mux/1
  Servo/1 -> Bus Selector/1
  Mux/1 -> Data Type Conversion1/1
  Data Type Conversion1/1 -> Servo_data/1  "Heading"
  Sensor/1 -> Bus Selector1/1
  Bus Selector1/1 -> Gain/1  "<quota_lidar>"
  Gain/1 -> Saturation/1
  Saturation/1 -> Mux/7

== system Aenea_model/AUTOPILOT_MODEL/AIR TX/Subsystem ==
  In1 : Inport
  In2 : Inport  Port=2
  Enable : EnablePort
  S-Function Builder : S-Function  FunctionName=MavLink_Send_sfun  SFunctionModules=MavLink_Send_sfun_wrapper  SFunctionDeploymentMode=off  EnableBusSupport=off  mask(S-Function Builder){}
      mask help: Simulink:masks:SFunctionBuilder_MD
      mask init: same as Aenea_model/LOG_DATA_MODEL/S-Function Builder
      settings: CopyFcn=set_param(gcbh,'LinkStatus','none')  OpenFcn=sfunctionwizard(gcbh)
      mask Display: plot(val(:,1),val(:,2)),disp(sys),port_label('input',1,'mavlink_buf_out'),port_label('input',2,'mavlink_buf_len')
  wires:
  In1/1 -> S-Function Builder/1
  In2/1 -> S-Function Builder/2

== system Aenea_model/AUTOPILOT_MODEL/AIR TX/SystemStatus ==
  note: coefficiente moltiplicativo Mavlink
  note: conversione
      | Amper - milliAmper
  note: NB.: se non si posside un dato inserire una costante con valore 0 (se non indicato diversamente sopra).
      | I dati vanno messi tutti anche se zeri nell'ordine elencato
  note: Vanno inseriti i collegamenti con i dati provenienti dal autopilota
      | in uscita bisogna dare 4 segnali:
      |
      | -onboard_control_sensor_present
      | - vettore con: load, voltaggio batteria(millivolt), drop rate, 5 flag di errore
      | -corrente della batteria (10*milliamper) -1 se non noto
      | -batteria rimanente (in percentuale) -1 se non noto
  note: conversione
      | Amper - milliAmper
  SyS_input : Inport
  Alarm : Inport  Port=2
  batteria : Inport  Port=3
  " " : Constant  Value=0  OutDataTypeStr=uint16
  Data Type Conversion : DataTypeConversion  OutDataTypeStr=uint32
  Data Type Conversion1 : DataTypeConversion  OutDataTypeStr=int16
  Data Type Conversion2 : DataTypeConversion  OutDataTypeStr=uint16
  Data Type Conversion3 : DataTypeConversion  OutDataTypeStr=int8
  Data Type Conversion4 : DataTypeConversion  OutDataTypeStr=uint16
  Demux : Demux  Outputs=3
  Gain : Gain  Gain=1000  OutDataTypeStr=uint16
  Gain1 : Gain  Gain=0.1  OutDataTypeStr=int16
  Gain2 : Gain  Gain=1000  OutDataTypeStr=int16
  Mux : Mux  Inputs=5
  load uint16 : Constant  Value=10  OutDataTypeStr=uint16
  onboard_control_sensor_present uint32 : Constant  Value=[1; 1 ;1]  OutDataTypeStr=uint32
  onboard : Outport  VectorParamsAs1DForOutWhenUnconnected=off
  LVDE : Outport  Port=2  VectorParamsAs1DForOutWhenUnconnected=off
  B_current : Outport  Port=3  VectorParamsAs1DForOutWhenUnconnected=off
  B_remaining : Outport  Port=4  VectorParamsAs1DForOutWhenUnconnected=off
  wires:
  Gain2/1 -> Gain1/1
  Demux/3 -> Gain2/1
  Gain1/1 -> Data Type Conversion1/1
  Demux/1 -> Gain/1
  batteria/1 -> Demux/1
  " "/1 -> Mux/4
  Data Type Conversion4/1 -> Mux/5
  Alarm/1 -> Data Type Conversion4/1
  SyS_input/1 -> Mux/3
  Data Type Conversion3/1 -> B_remaining/1  "B_Remaining"
  Data Type Conversion1/1 -> B_current/1  "B_Current"
  Data Type Conversion2/1 -> LVDE/1  "LVDE"
  Data Type Conversion/1 -> onboard/1  "onboard"
  Demux/2 -> Data Type Conversion3/1
  Mux/1 -> Data Type Conversion2/1
  Gain/1 -> Mux/2
  load uint16/1 -> Mux/1
  onboard_control_sensor_present uint32/1 -> Data Type Conversion/1

== system Aenea_model/AUTOPILOT_MODEL/AIR TX/VFR ==
  note: NB.: se non si posside un dato inserire una costante con valore 0. I dati vanno messi tutti anche se zeri nell'ordine elencato
  note: Vanno inseriti i collegamenti con i dati provenienti dal sensore di velocità
      | in uscita bisogna dare 3 segnali:
      |
      | -  AGAC: airspeed, groundspeed,altitudine, rateo salita
      | -Heading
      | -Throttle: spinta o rpm del motore
  note: inserire 100/massimo valore
      | deve uscire una percentuale
      | FISSATO PER QUOTA IL 5-5-2016
  VFR1 : Inport
  Bus Selector : BusSelector  OutputSignals=ias,Alt,RC,heading,RPM
  Data Type Conversion : DataTypeConversion  OutDataTypeStr=single
  Data Type Conversion1 : DataTypeConversion  OutDataTypeStr=int16  RndMeth=Simplest
  Data Type Conversion2 : DataTypeConversion  OutDataTypeStr=uint16  RndMeth=Simplest
  Mux : Mux
  Radians to Degrees : simulink_extras/Transformations/Radians to Degrees
  USCITA PERCENTUALE : Gain  Gain=100/9000
  airspeed groundspeed alt climb1 : Constant  Value=0  OutDataTypeStr=double  SampleTime=t_AP
  wrapTo360 : Subsystem
  AGAC : Outport  VectorParamsAs1DForOutWhenUnconnected=off
  Heading : Outport  Port=2  VectorParamsAs1DForOutWhenUnconnected=off
  Throttle : Outport  Port=3  VectorParamsAs1DForOutWhenUnconnected=off
  wires:
  Mux/1 -> Data Type Conversion/1
  Bus Selector/5 -> USCITA PERCENTUALE/1  "<RPM>"
  Bus Selector/4 -> Radians to Degrees/1  "<heading>"
  Bus Selector/3 -> Mux/4  "<RC>"
  Bus Selector/2 -> Mux/3  "<Alt>"
  Bus Selector/1 -> Mux/1  "<ias>"
  airspeed groundspeed alt climb1/1 -> Mux/2
  VFR1/1 -> Bus Selector/1
  Data Type Conversion2/1 -> Throttle/1  "Throttle"
  Data Type Conversion1/1 -> Heading/1  "Heading"
  Data Type Conversion/1 -> AGAC/1  "AGAC"
  USCITA PERCENTUALE/1 -> Data Type Conversion2/1
  Radians to Degrees/1 -> wrapTo360/1(In1)
  wrapTo360/1(Out1) -> Data Type Conversion1/1  "uscita"

== system Aenea_model/AUTOPILOT_MODEL/AIR TX/Waypoints ==
  GC_req : Inport
  "Sensori " : Inport  Port=2
  Bus Selector : BusSelector  OutputSignals=Alt
  Bus Selector3 : BusSelector  OutputSignals=Val_float,WP_db_info,WP_db_param,GC_info
  MATLAB Function : MATLAB Function  TreatAsAtomicUnit=on
  Terminator : Terminator
  GC_info : Outport  VectorParamsAs1DForOutWhenUnconnected=off
  P_value : Outport  Port=2  VectorParamsAs1DForOutWhenUnconnected=off
  WP_info : Outport  Port=3  VectorParamsAs1DForOutWhenUnconnected=off
  WP_param : Outport  Port=4  VectorParamsAs1DForOutWhenUnconnected=off
  wires:
  "Sensori "/1 -> Bus Selector/1
  Bus Selector3/1 -> P_value/1  "<Val_float>"
  Bus Selector/1 -> Terminator/1  "<Alt>"
  MATLAB Function/2(WP_param) -> WP_param/1
  Bus Selector3/3 -> MATLAB Function/2(WP_param_in)  "<WP_db_param>"
  MATLAB Function/1(WP_info) -> WP_info/1
  Bus Selector3/2 -> MATLAB Function/1(WP_info_in)  "<WP_db_info>"
  Bus Selector3/4 -> MATLAB Function/3(GC_info), GC_info/1  "<GC_info>"
  GC_req/1 -> Bus Selector3/1

== system Aenea_model/AUTOPILOT_MODEL/AUTOPILOTA/AUTOPILOTI1 ==
  Sensori : Inport
  Parametri Sistema di Controllo : Inport  Port=2
  Riferimenti : Inport  Port=3
  Riferimenti Safe : Inport  Port=4
  Alarm Safe : Inport  Port=5
  comandi : Inport  Port=6
  Switch attuatori : Inport  Port=7
  Switch_ATO : Inport  Port=8
  Switch_AL : Inport  Port=9
  traking theta : Inport  Port=10
  manetta_track : Inport  Port=11
  track_phi : Inport  Port=12
  Bus Creator : BusCreator  Inputs=2
  Bus Selector : BusSelector  OutputSignals=switch_manetta,switch_alettoni
  Bus Selector2 : BusSelector  OutputSignals=throttle_safe,theta_safe,phi_safe
  CONTROLLORE DI QUOTA : Subsystem
  CONTROLLORE DI ROTTA : Subsystem
  CONTROLLORE DI VELOCITA' : Subsystem
  Switch di selezione riferimeti per i loop interni 1 : MultiPortSwitch  DataPortOrder=Zero-based contiguous  Inputs=2  zeroidx=on
  Switch di selezioneriferimeti per i loop interni 2 : MultiPortSwitch  DataPortOrder=Zero-based contiguous  Inputs=2  zeroidx=on
  Switch di selezioneriferimeti per i loop interni 3 : MultiPortSwitch  DataPortOrder=Zero-based contiguous  Inputs=2  zeroidx=on
  Riferimento Manetta : Outport  VectorParamsAs1DForOutWhenUnconnected=off
  Riferimenti Rollio e Beccheggio : Outport  Port=2  VectorParamsAs1DForOutWhenUnconnected=off
  tag scope: alarm_safe=global, phi_safe=global, theta_safe=global, throttle_safe=global
  wires:
  Bus Creator/1 -> Riferimenti Rollio e Beccheggio/1  "Rif_loop_int"
  CONTROLLORE DI VELOCITA'/1(Riferimento Manetta) -> Switch di selezione riferimeti per i loop interni 1/2  "Riferimento Manetta"
  Switch di selezione riferimeti per i loop interni 1/1 -> Riferimento Manetta/1  "Riferimento Manetta"
  Switch di selezioneriferimeti per i loop interni 2/1 -> Bus Creator/1  "theta_rif"
  Switch di selezioneriferimeti per i loop interni 3/1 -> Bus Creator/2  "phi_rif"
  [alarm_safe] -> Switch di selezioneriferimeti per i loop interni 2/1
  [alarm_safe] -> Switch di selezioneriferimeti per i loop interni 3/1
  Sensori/1 -> CONTROLLORE DI VELOCITA'/1(Sensori), CONTROLLORE DI ROTTA/2(Sensori), CONTROLLORE DI QUOTA/1(Sensori)
  Riferimenti/1 -> CONTROLLORE DI ROTTA/1(Riferimenti), CONTROLLORE DI QUOTA/2(Riferimenti), CONTROLLORE DI VELOCITA'/2(Riferimenti)
  Parametri Sistema di Controllo/1 -> CONTROLLORE DI VELOCITA'/3(Parametri Sistema di Controllo), CONTROLLORE DI QUOTA/3(Parametri Sistema di Controllo), CONTROLLORE DI ROTTA/3(Parametri Sistema di Controllo)
  Riferimenti Safe/1 -> Bus Selector2/1
  Alarm Safe/1 -> [alarm_safe]
  Bus Selector2/1 -> [throttle_safe]  "<throttle_safe>"
  Bus Selector2/2 -> [theta_safe]  "<theta_safe>"
  Bus Selector2/3 -> [phi_safe]  "<phi_safe>"
  [alarm_safe] -> Switch di selezione riferimeti per i loop interni 1/1
  [throttle_safe] -> Switch di selezione riferimeti per i loop interni 1/3
  [theta_safe] -> Switch di selezioneriferimeti per i loop interni 2/3
  [phi_safe] -> Switch di selezioneriferimeti per i loop interni 3/3
  Switch attuatori/1 -> Bus Selector/1
  Bus Selector/1 -> [switch_manetta]  "<switch_manetta>"
  Bus Selector/2 -> [switch_alettoni]  "<switch_alettoni>"
  comandi/1 -> CONTROLLORE DI VELOCITA'/5(comandi)
  [switch_manetta] -> CONTROLLORE DI VELOCITA'/4(switch_manetta)
  [switch_alettoni] -> CONTROLLORE DI ROTTA/4("switch alettoni ")
  CONTROLLORE DI ROTTA/1(phi_rif) -> Switch di selezioneriferimeti per i loop interni 3/2  "phi_rif"
  Switch_ATO/1 -> [Switch_ATO]
  Switch_AL/1 -> [Switch_AL]
  [Switch_AL] -> CONTROLLORE DI VELOCITA'/6(Switch_AL)
  CONTROLLORE DI QUOTA/1(theta_rif) -> Switch di selezioneriferimeti per i loop interni 2/2  "theta_rif"
  [Switch_ATO] -> CONTROLLORE DI QUOTA/4(Ato)
  traking theta/1 -> CONTROLLORE DI QUOTA/5(traking_theta)
  manetta_track/1 -> CONTROLLORE DI VELOCITA'/7(manetta_track)
  track_phi/1 -> CONTROLLORE DI ROTTA/5(track_phi)
  [Switch_ATO] -> CONTROLLORE DI ROTTA/6(Switch_ATO)

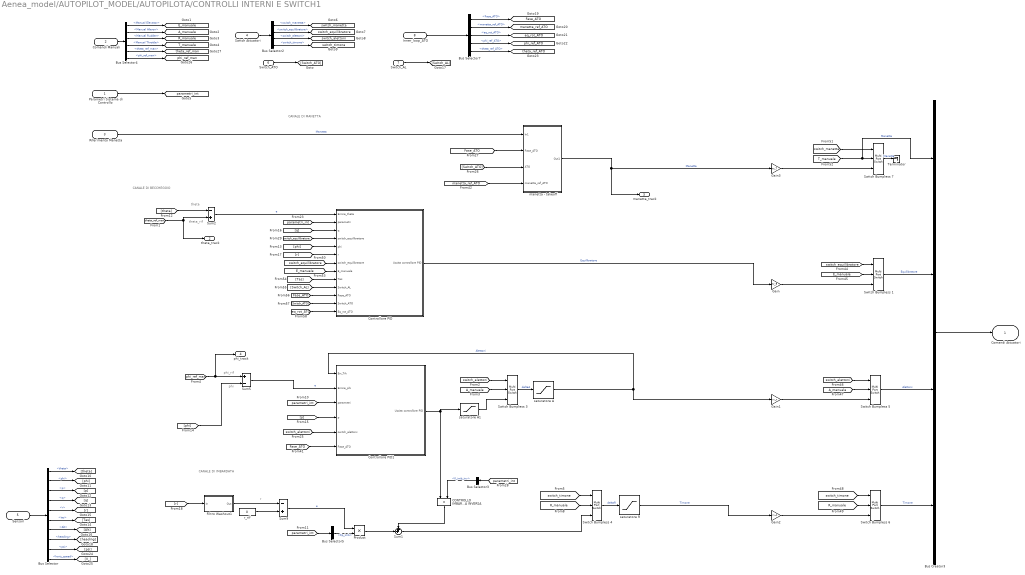
== system Aenea_model/AUTOPILOT_MODEL/AUTOPILOTA/CONTROLLI INTERNI E SWITCH1 ==
  note: CANALE DI
      |  MANETTA
  note: theta
  note: theta_rif
  note: CANALE DI
      |  BECCHEGGIO
  note: CANALE
      | DI IMBARDATA
  note: phi
  note: phi_rif
  note: r
  Parametri Sistema di Controllo : Inport
  Comandi Manuali : Inport  Port=2
  Riferimento Manetta : Inport  Port=3
  Switch Attuatori : Inport  Port=4
  Sensori : Inport  Port=5
  Switch_ATO : Inport  Port=6
  Switch_AL : Inport  Port=7
  Inner_loop_ATO : Inport  Port=8
  "  CONTROLLO IMBARDATA INVERSA" : Product  RndMeth=Zero
  Bus Creator3 : BusCreator  Inputs=4
  Bus Selector : BusSelector  OutputSignals=theta,phi,p,q,r,ias,Alt,heading,psi,horiz_speed
  Bus Selector2 : BusSelector  OutputSignals=switch_manetta,switch_equilibratore,switch_alettoni,switch_timone
  Bus Selector3 : BusSelector  OutputSignals=K_imb_inv
  Bus Selector4 : BusSelector  OutputSignals=Manual Elevator,Manual Aileron,Manual Rudder,Manual Throttle,theta_ref_man,phi_ref_man
  Bus Selector5 : BusSelector  OutputSignals=Kp_imb
  Bus Selector7 : BusSelector  OutputSignals=Fase_ATO,manetta_ref_ATO,eq_rot_ATO,phi_ref_ATO,theta_ref_ATO
  Controllore PID : Subsystem
  Controllore PID1 : Subsystem
  Filtro Washout1 : Subsystem
  Gain : Gain  Gain=inv_E
  Gain1 : Gain  Gain=inv_A
  Gain2 : Gain  Gain=inv_R
  Gain3 : Gain  Gain=inv_T
  Product : Product  RndMeth=Zero
  Sum1 : Sum  Inputs=++|
  Sum2 : Sum  Inputs=-+
  Sum5 : Sum  Inputs=+-
  Sum9 : Sum  Inputs=-+
  Switch Bumpless {1,3..7} (6 alike) : MultiPortSwitch  DataPortOrder=Zero-based contiguous  Inputs=2  zeroidx=on
  Terminator : Terminator
  manetta - takeoff : Subsystem
  r_rif : Constant  Value=0
  saturatore A : Saturate  UpperLimit=attuatore_Amax  LowerLimit=attuatore_Amin
  saturatore A1 : Saturate  UpperLimit=attuatore_Amax  LowerLimit=attuatore_Amin
  saturatore R : Saturate  UpperLimit=attuatore_Rmax  LowerLimit=attuatore_Rmin
  Comandi Attuatori : Outport  VectorParamsAs1DForOutWhenUnconnected=off
  theta_track : Outport  Port=2  VectorParamsAs1DForOutWhenUnconnected=off
  manetta_track : Outport  Port=3  VectorParamsAs1DForOutWhenUnconnected=off
  phi_track : Outport  Port=4  VectorParamsAs1DForOutWhenUnconnected=off
  tag scope: A_manuale=global, E_manuale=global, Fase_ATO=global, R_manuale=global, T_manuale=global, eq_rot_ATO=global, manetta_ref_ATO=global, parametri_int=global, phi_ref_ATO=global, phi_ref_man=global, switch_alettoni=global, switch_equilibratore=global, switch_manetta=global, switch_timone=global, theta_ref_ATO=global, theta_ref_man=global
  wires:
  Comandi Manuali/1 -> Bus Selector4/1
  Bus Selector4/1 -> [E_manuale]  "<Manual Elevator>"
  Bus Selector4/2 -> [A_manuale]  "<Manual Aileron>"
  Bus Selector4/3 -> [R_manuale]  "<Manual Rudder>"
  Bus Selector4/4 -> [T_manuale]  "<Manual Throttle>"
  Parametri Sistema di Controllo/1 -> [parametri_int]
  Switch Attuatori/1 -> Bus Selector2/1
  Bus Selector2/1 -> [switch_manetta]  "<switch_manetta>"
  Bus Selector2/2 -> [switch_equilibratore]  "<switch_equilibratore>"
  Bus Selector2/3 -> [switch_alettoni]  "<switch_alettoni>"
  Bus Selector2/4 -> [switch_timone]  "<switch_timone>"
  Sensori/1 -> Bus Selector/1
  Switch Bumpless 3/1 -> saturatore A/1  "deltaA"
  saturatore A/1 -> Gain1/1, Controllore PID1/1(Err_Trk)  "Alettoni"
  [switch_alettoni] -> Switch Bumpless 3/1
  [A_manuale] -> Switch Bumpless 3/2
  [switch_timone] -> Switch Bumpless 4/1
  [R_manuale] -> Switch Bumpless 4/2
  r_rif/1 -> Sum9/2
  Filtro Washout1/1(Out) -> Sum9/1
  Bus Creator3/1 -> Comandi Attuatori/1
  Bus Selector3/1 -> "  CONTROLLO IMBARDATA INVERSA"/2  "<K_imb_inv>"
  [parametri_int] -> Bus Selector3/1
  Sum2/1 -> Controllore PID/1(Errore_theta)  "e"
  [switch_equilibratore] -> Controllore PID/4("switch_equilibratore ")
  saturatore A1/1 -> Switch Bumpless 3/3
  [parametri_int] -> Controllore PID/2(parametri)
  [parametri_int] -> Controllore PID1/3(parametri)
  Sum5/1 -> Controllore PID1/2(Errore_phi)  "e"
  Controllore PID1/1(Uscita controllore PID) -> saturatore A1/1, "  CONTROLLO IMBARDATA INVERSA"/1
  saturatore R/1 -> Gain2/1  "Timone"
  Switch Bumpless 4/1 -> saturatore R/1  "deltaR"
  Sum9/1 -> Product/1  "e"
  [parametri_int] -> Bus Selector5/1
  Bus Selector5/1 -> Product/2  "<Kp_imb>"
  Product/1 -> Sum1/2
  "  CONTROLLO IMBARDATA INVERSA"/1 -> Sum1/1
  Switch_ATO/1 -> [Switch_ATO]
  Bus Selector/6 -> [Tas]  "<ias>"
  Bus Selector/7 -> [Alt]  "<Alt>"
  Sum1/1 -> Switch Bumpless 4/3
  Switch_AL/1 -> [Switch_AL]
  Controllore PID/1(Uscita controllore PID) -> Gain/1  "Equilibratore"
  [phi_ref_man] -> phi_track/1, Sum5/1
  Inner_loop_ATO/1 -> Bus Selector7/1
  Bus Selector7/1 -> [Fase_ATO]  "<Fase_ATO>"
  Bus Selector7/2 -> [manetta_ref_ATO]  "<manetta_ref_ATO>"
  Bus Selector7/3 -> [eq_rot_ATO]  "<eq_rot_ATO>"
  Bus Selector7/4 -> [phi_ref_ATO]  "<phi_ref_ATO>"
  Bus Selector7/5 -> [theta_ref_ATO]  "<theta_ref_ATO>"
  manetta - takeoff/1(Out1) -> Gain3/1, manetta_track/1  "Manetta"
  Riferimento Manetta/1 -> manetta - takeoff/1(In1)  "Manetta"
  [switch_alettoni] -> Controllore PID1/5("switch_alettoni ")
  [theta] -> Sum2/1
  Bus Selector/1 -> [theta]  "<theta>"
  [phi] -> Controllore PID/5("phi ")
  [phi] -> Sum5/2
  Bus Selector/2 -> [phi]  "<phi>"
  [p] -> Controllore PID1/4("p ")
  Bus Selector/3 -> [p]  "<p>"
  [q] -> Controllore PID/3("q ")
  Bus Selector/4 -> [q]  "<q>"
  [r] -> Controllore PID/6(r)
  [r] -> Filtro Washout1/1(In)
  Bus Selector/5 -> [r]  "<r>"
  Bus Selector/9 -> [psi]  "<psi>"
  [Switch_ATO] -> manetta - takeoff/3(ATO)
  [Fase_ATO] -> manetta - takeoff/2(Fase_ATO)
  [manetta_ref_ATO] -> manetta - takeoff/4(manetta_ref_ATO)
  [Fase_ATO] -> Controllore PID1/6(Fase_ATO)
  Bus Selector/8 -> [heading]  "<heading>"
  Bus Selector/10 -> [V_]  "<horiz_speed>"
  Switch Bumpless 1/1 -> Bus Creator3/2  "Equilibratore"
  [E_manuale] -> Switch Bumpless 1/2
  [switch_equilibratore] -> Switch Bumpless 1/1
  Gain/1 -> Switch Bumpless 1/3
  [switch_alettoni] -> Switch Bumpless 5/1
  [A_manuale] -> Switch Bumpless 5/2
  Switch Bumpless 5/1 -> Bus Creator3/3  "Alettoni"
  Gain1/1 -> Switch Bumpless 5/3
  [switch_timone] -> Switch Bumpless 6/1
  [R_manuale] -> Switch Bumpless 6/2
  Switch Bumpless 6/1 -> Bus Creator3/4  "Timone"
  Gain2/1 -> Switch Bumpless 6/3
  [switch_manetta] -> Switch Bumpless 7/1
  [T_manuale] -> Bus Creator3/1, Switch Bumpless 7/2  "Manetta"
  Gain3/1 -> Switch Bumpless 7/3
  [switch_equilibratore] -> Controllore PID/7(switch_equilibratore)
  [E_manuale] -> Controllore PID/8(E_manuale)
  [Switch_AL] -> Controllore PID/10(Switch_AL)
  [Tas] -> Controllore PID/9(Tas)
  [Fase_ATO] -> Controllore PID/11(Fase_ATO)
  [Switch_ATO] -> Controllore PID/12(Switch_ATO)
  [eq_rot_ATO] -> Controllore PID/13(Eq_rot_ATO)
  Bus Selector4/6 -> [phi_ref_man]  "<phi_ref_man>"
  Bus Selector4/5 -> [theta_ref_man]  "<theta_ref_man>"
  [theta_ref_man] -> Sum2/2, theta_track/1
  Switch Bumpless 7/1 -> Terminator/1  "Manetta"
